simulink model "SC_PID_eval"  (R2021a)
settings: Solver=FixedStepAuto  StartTime=0.0  StopTime=T  FixedStep=Ts  MaxStep=0.1  RelTol=1e-3  EnableMultiTasking=on
PreLoadFcn:
  | K=10.8;
  | TI=2.56;
  | TD=0;
  | u=0;
InitFcn:
  | seed = randi(10000);
StartFcn:
  | seed = randi(10000);
libraries: simulink_extras x2, simulink_need_slupdate x1
settings Model: Creator=jiaya  LastModifiedBy=jiaya
settings SolverCC: AlgebraicLoopSolver=TrustRegion
settings DataIOCC: LimitDataPoints=on  SaveFormat=Array  SignalLoggingSaveFormat=ModelDataLogs  ReturnWorkspaceOutputs=off
settings OptimizationCC: InitFltsAndDblsToZero=on  LifeSpan=inf
settings DebuggingCC: SaveWithParameterizedLinksMsg=none  UnderspecifiedInitializationDetection=Classic  MergeDetectMultiDrivingBlocksExec=none  SignalResolutionControl=TryResolveAllWithWarning  MultiTaskDSMMsg=warning  MultiTaskCondExecSysMsg=none  FcnCallInpInsideContextMsg=warning  SFUnexpectedBacktrackingDiag=warning  SFNoUnconditionalDefaultTransitionDiag=warning  SFExecutionAtInitializationDiag=none  SFMachineParentedDataDiag=warning  ArithmeticOperatorsInVariantConditions=warning
settings HardwareCC: ProdBitPerPointer=32  ProdBitPerSizeT=32  ProdBitPerPtrDiffT=32  ProdLargestAtomicFloat=None  ProdIntDivRoundTo=Undefined  ProdEndianess=Unspecified  ProdWordSize=32  ProdHWDeviceType=32-bit Generic  TargetUnknown=on
settings ModelReferenceCC: PropagateSignalLabelsOutOfModel=off
settings CodeAppCC: StateflowObjectComments=on
settings GRTTargetCC: TargetFcnLib=ansi_tfl_tmw.mat  TargetLangStandard=C89/C90 (ANSI)  CombineOutputUpdateFcns=off  GRTInterface=on
settings ConfigComp: CovMetricSettings=dw  CovSaveCumulativeToWorkspaceVar=on  CovSaveSingleToWorkspaceVar=on

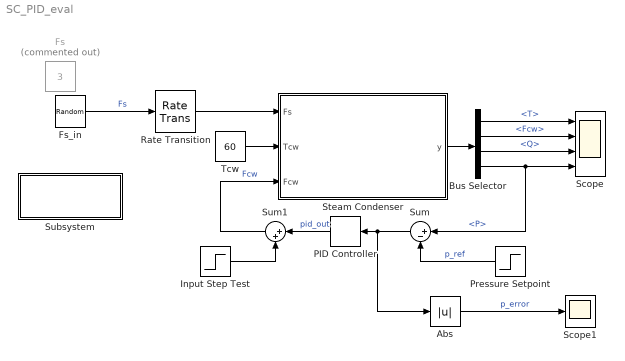
== system SC_PID_eval ==
  Abs : Abs
  Bus Selector : BusSelector  OutputSignals=T,Fcw,Q,P
  Fs : Constant  Commented=on  Value=3
  Fs_in : UniformRandomNumber  Minimum=3.99  Maximum=4.01  Seed=seed  SampleTime=5  VectorParams1D=off
  Input Step Test : Step  Time=10  After=u  SampleTime=0
  PID Controller : simulink_need_slupdate/PID Controller  P=K  I=K/TI  D=TD
  Pressure Setpoint : Step  Time=2  Before=90  After=87  SampleTime=0
  Rate Transition : RateTransition  OutPortSampleTime=Ts
  Scope : Scope  NumInputPorts=4
  Scope1 : Scope
  Steam Condenser : Subsystem  mask{V=3, Mcw=500, UA=356.972413581334, tau=1, Fcw=107.8880952381, P=90, T=80}
      mask prompts: V "Volume [m3]"; Mcw "CW Holdup [kg]"; UA "UA [kW/K]"; tau "Actuator time constant [s]"; Fcw "Fcw [kg/s]"; P "P [kPa]"; T "T [degC]"
      mask init:
      | y1=[.3 .3 .7 .7 .3 NaN .4 .4 NaN .5 .5 NaN .6 .6 NaN 0.2 0.3 NaN 0.7 0.8 NaN 0.7 0.8 NaN 0.82 NaN 0.18];
      | x1=[.8 .2 .2 .8 .8 NaN .8 .2 NaN .8 .2 NaN .8 .2 NaN 0.5 0.5 NaN 0.3 0.3 NaN 0.7 0.7 NaN -0.05 NaN 1.05];
      | y2=0.3:0.05:0.7;
      | x2=sqrt(0.0625-(y2-0.5).^2);
      | y3=[.5 .5 .8 NaN 0.2 0.4 0.4];
      | x3=[x2(5)+0.65 0.95 0.95 NaN .1 .1 0.35-x2(3)];
      mask Display:
      | plot([x1 NaN 0.65+x2 NaN 0.35-x2 NaN x3],[y1 NaN y2 NaN y2 NaN y3])
      | port_label('input',1,'Fs')
      | port_label('input',2,'Tcw')
      | port_label('input',3,'Fcw')
      | port_label('output',1,'y')
  Subsystem : Subsystem
      settings: OpenFcn=|
      | K=0;TI=1;TD=0;u=1;
      | sim('SteamCondenser')
      | [Kp,tau,td]=ReactionCurve(y.time,y.signals(4).values);
      | td=td-10;
      | K=-(0.9/Kp)*(tau/td);
      | TI=3.3*td;
      | u=0;
      | sim('SteamCondenser')
      mask Display: disp(sprintf('Reaction Curve\n PID Tuning'))
  Sum : Sum  Inputs=|+-  InputSameDT=on  OutDataTypeStr=Inherit: Same as first input
  Sum1 : Sum  Inputs=|++  InputSameDT=on  OutDataTypeStr=Inherit: Same as first input
  Tcw : Constant  Value=60  VectorParams1D=off
  wires:
  Steam Condenser/1(y) -> Bus Selector/1
  Tcw/1 -> Steam Condenser/2(Tcw)
  Pressure Setpoint/1 -> Sum/2  "p_ref"
  Bus Selector/1 -> Scope/1  "<T>"
  Bus Selector/2 -> Scope/2  "<Fcw>"
  Bus Selector/3 -> Scope/3  "<Q>"
  Bus Selector/4 -> Sum/1, Scope/4  "<P>"
  PID Controller/1 -> Sum1/1  "pid_out"
  Sum1/1 -> Steam Condenser/3(Fcw)  "Fcw"
  Input Step Test/1 -> Sum1/2
  Rate Transition/1 -> Steam Condenser/1(Fs)
  Fs_in/1 -> Rate Transition/1  "Fs"
  Abs/1 -> Scope1/1  "p_error"
  Sum/1 -> Abs/1, PID Controller/1

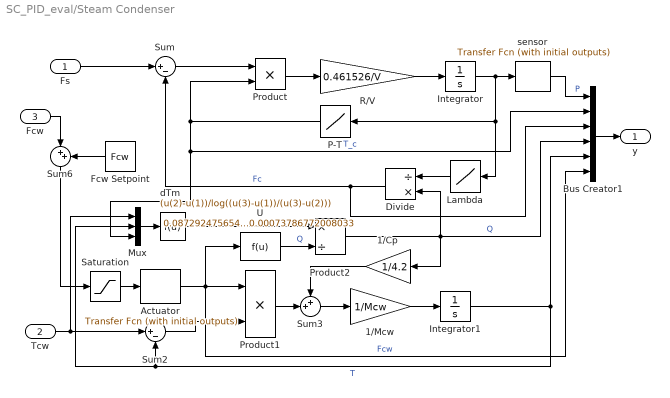
== system SC_PID_eval/Steam Condenser ==
  Fs : Inport
  Tcw : Inport  Port=2
  Fcw : Inport  Port=3
  1/Cp : Gain  Gain=1/4.2  OutDataTypeStr=Inherit: Same as input  ParamDataTypeStr=Inherit: Same as input
  1/Mcw : Gain  Gain=1/Mcw  OutDataTypeStr=Inherit: Same as input  ParamDataTypeStr=Inherit: Same as input
  Actuator : simulink_extras/Additional Linear/Transfer Fcn (with initial outputs)  N=[1]  D=[tau 1]  Y0=Fcw  U0=Fcw
  Bus Creator1 : BusCreator  Inputs=6
  Divide : Product  Inputs=/*  InputSameDT=on  RndMeth=Zero  OutDataTypeStr=Inherit: Same as first input
  Fcw Setpoint : Constant  Value=Fcw
  Integrator : Integrator  InitialCondition=P
  Integrator1 : Integrator  InitialCondition=T
  Lambda : Lookup  InputValues=[50 60 70 80 90 100 110]  Table=[2305.42 2293.64 2283.30 2274.05 2265.65 2257.92 2250.76]  SaturateOnIntegerOverflow=on
  Mux : Mux  Inputs=3
  P-T : Lookup  InputValues=[50 60 70 80 90 100 110]  Table=[81.3167 85.9258 89.9315 93.4854 96.6870 99.6059 102.2923]  SaturateOnIntegerOverflow=on
  Product : Product  InputSameDT=on  RndMeth=Zero  OutDataTypeStr=Inherit: Same as first input
  Product1 : Product  InputSameDT=on  RndMeth=Zero  OutDataTypeStr=Inherit: Same as first input
  Product2 : Product  Inputs=*/  InputSameDT=on  RndMeth=Zero  OutDataTypeStr=Inherit: Same as first input
  R/V : Gain  Gain=0.461526/V  OutDataTypeStr=Inherit: Same as input  ParamDataTypeStr=Inherit: Same as input
  Saturation : Saturate  UpperLimit=200  LowerLimit=0
  Sum : Sum  Inputs=|+-  InputSameDT=on  OutDataTypeStr=Inherit: Same as first input
  Sum2 : Sum  Inputs=|+-  InputSameDT=on  OutDataTypeStr=Inherit: Same as first input
  Sum3 : Sum  Inputs=++|  InputSameDT=on  OutDataTypeStr=Inherit: Same as first input
  Sum6 : Sum  Inputs=|++  InputSameDT=on  OutDataTypeStr=Inherit: Same as first input
  U : Fcn  Expr=0.0872924756541668/u^0.8+0.00073786772008033
  dTm : Fcn  Expr=(u(2)-u(1))/log((u(3)-u(1))/(u(3)-u(2)))
  sensor : simulink_extras/Additional Linear/Transfer Fcn (with initial outputs)  N=[1]  D=[tau/2 1]  Y0=P  U0=P
  y : Outport
  wires:
  R/V/1 -> Integrator/1
  Product/1 -> R/V/1
  Sum/1 -> Product/1
  Fs/1 -> Sum/1
  Integrator/1 -> sensor/1, Lambda/1, P-T/1
  1/Mcw/1 -> Integrator1/1
  Integrator1/1 -> Sum2/2, Mux/2, Bus Creator1/5  "T"
  Tcw/1 -> Sum2/1, Mux/1
  Sum2/1 -> Product1/2
  Product1/1 -> Sum3/2
  Sum3/1 -> 1/Mcw/1
  1/Cp/1 -> Sum3/1
  dTm/1 -> Product2/1
  Bus Creator1/1 -> y/1
  Actuator/1 -> Product1/1, U/1, Bus Creator1/6  "Fcw"
  sensor/1 -> Bus Creator1/1  "P"
  Saturation/1 -> Actuator/1
  Sum6/1 -> Saturation/1
  Fcw/1 -> Sum6/1
  Fcw Setpoint/1 -> Sum6/2
  Lambda/1 -> Divide/1
  Divide/1 -> Sum/2, Bus Creator1/3  "Fc"
  P-T/1 -> Product/2, Mux/3, Bus Creator1/2  "T_c"
  Mux/1 -> dTm/1
  Product2/1 -> 1/Cp/1, Divide/2, Bus Creator1/4  "Q"
  U/1 -> Product2/2  "Q"

== system SC_PID_eval/Subsystem ==
